simulink model "OS"  (R2024a)
settings: Solver=FixedStepDiscrete  StartTime=0.0  StopTime=10.0  FixedStep=0.5  RelTol=1e-3
settings Model: Creator=VICTUS  LastModifiedBy=VICTUS

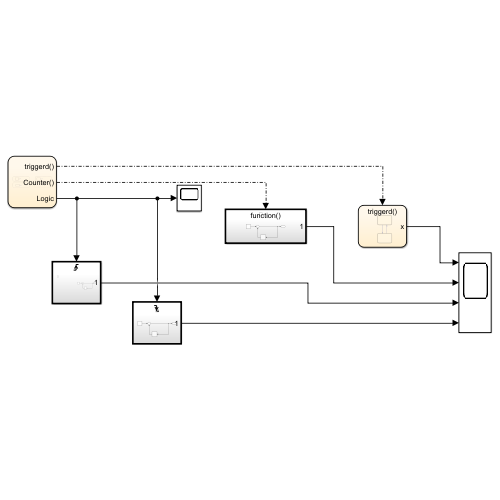
[thumbnail: Simulink's stored preview of the top-level diagram]
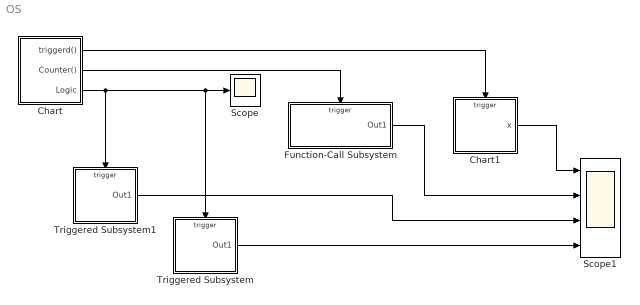
== system OS ==
  Chart : Stateflow chart  TreatAsAtomicUnit=on
  Chart1 : Stateflow chart  TreatAsAtomicUnit=on
  Function-Call Subsystem : Subsystem  TreatAsAtomicUnit=on
  Scope : Scope
  Scope1 : Scope  NumInputPorts=4
  Triggered Subsystem : Subsystem  TreatAsAtomicUnit=on
  Triggered Subsystem1 : Subsystem  TreatAsAtomicUnit=on
  wires:
  Chart/1(triggerd()) -> Chart1/Trigger
  Chart/2(Counter()) -> Function-Call Subsystem/Trigger
  Chart/3(Logic) -> Scope/1, Triggered Subsystem/Trigger, Triggered Subsystem1/Trigger
  Function-Call Subsystem/1(Out1) -> Scope1/2
  Triggered Subsystem/1(Out1) -> Scope1/4
  Triggered Subsystem1/1(Out1) -> Scope1/3
  Chart1/1(x) -> Scope1/1

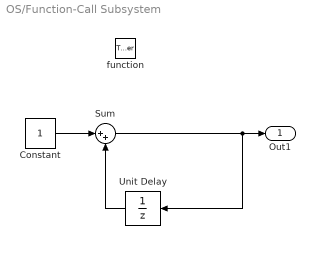
== system OS/Function-Call Subsystem ==
  function : TriggerPort  TriggerType=function-call  VariantControl=(inherit)
  Constant : Constant
  Sum : Sum  Inputs=|++
  Unit Delay : UnitDelay  SampleTime=-1  HasFrameUpgradeWarning=on
  Out1 : Outport
  wires:
  Sum/1 -> Out1/1, Unit Delay/1
  Unit Delay/1 -> Sum/2
  Constant/1 -> Sum/1

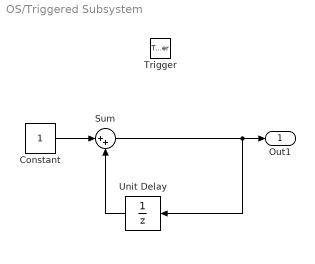
== system OS/Triggered Subsystem ==
  Trigger : TriggerPort  TriggerType=falling  VariantControl=(inherit)
  Constant : Constant
  Sum : Sum  Inputs=|++
  Unit Delay : UnitDelay  SampleTime=-1  HasFrameUpgradeWarning=on
  Out1 : Outport
  wires:
  Sum/1 -> Out1/1, Unit Delay/1
  Constant/1 -> Sum/1
  Unit Delay/1 -> Sum/2

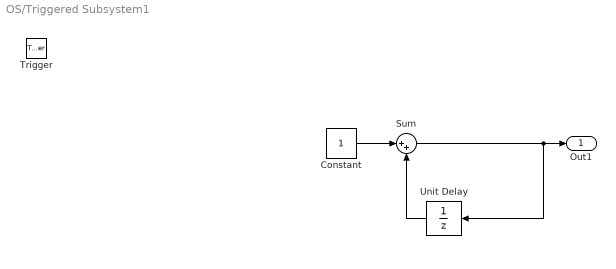
== system OS/Triggered Subsystem1 ==
  Trigger : TriggerPort  VariantControl=(inherit)
  Constant : Constant
  Sum : Sum  Inputs=|++
  Unit Delay : UnitDelay  SampleTime=-1  HasFrameUpgradeWarning=on
  Out1 : Outport
  wires:
  Sum/1 -> Out1/1, Unit Delay/1
  Constant/1 -> Sum/1
  Unit Delay/1 -> Sum/2

== stateflow chart OS/Chart1 ==
  state S1
    en:
    x = 0;
  state S2
    en:
    x=1;
  (default) -> S1
  S1 -> S2 : triggerd
  S2 -> S1 : triggerd
  data: x output
  events: triggerd input FUNCTION_CALL_EVENT

== stateflow chart OS/Chart ==
  state S1 [parallel]
    settings: executionOrder=1
    state A
    A -> A : after(0.5,sec)/{triggerd}
  state S2 [parallel]
    settings: executionOrder=2
    state B
    B -> B : after(1,sec)/{Counter}
  state S3 [parallel]
    settings: executionOrder=3
    state C
    C -> C : after(1.5,sec)/{Logic}
  state S4 [parallel] [commented out]
    state D [commented out]
    D -> D [commented out]
  events: triggerd output FUNCTION_CALL_EVENT; Counter output FUNCTION_CALL_EVENT; Logic output EITHER_EDGE_EVENT
